simulink model "Boeing787_OldMission_ElectricalThermalHydraulicFuelECS"  (R2013a)
settings: Solver=ode23tb  SolverMode=SingleTasking  StartTime=0.0  StopTime=346  RelTol=1e-3
InitFcn:
  | load('SampleOutput.mat')
  | 
  | load('SampleFuelBurn.mat')
undefined symbols (not defined in the file or in its folder): ailerons, AirProp, B_737, elevator, FuelBurn, HydProp, landing_gear, rudder, thrust_rev
libraries: PowerFlowLib x118, simulink x20
(part 17 of 26)

== system Boeing787_OldMission_ElectricalThermalHydraulicFuelECS/Fuel ==
  note: Fuel & Oil System
  ECS : Inport
  Eng1 : Inport  Port=2
  Eng2 : Inport  Port=3  PortDimensions=11
  Bus Creator : BusCreator  Inputs=3
  Constant : Constant  Value=50
  Constant1 : Constant  Value=1700
  Constant2 : Constant  Value=1700
  Constant{3..6} (4 alike) : Constant  Value=0
  ElectricalSink : PowerFlowLib/Support Functions//Tools/ElectricalSink  Tag=Flow  Description=TwoPhase  load_loc=Empennage  ACDC_load=AC  units=Kilowatts  unq_id=2143
  ElectricalSink1 : PowerFlowLib/Support Functions//Tools/ElectricalSink  Tag=Flow  Description=TwoPhase  load_loc=Cagobay  ACDC_load=AC  units=Kilowatts  unq_id=9219
  ElectricalSink2 : PowerFlowLib/Support Functions//Tools/ElectricalSink  Tag=Flow  Description=TwoPhase  load_loc=Cabin  ACDC_load=AC  units=Kilowatts  unq_id=6691
  Fuel Tanks/Pumps : Subsystem
  Heat Exchanger : PowerFlowLib/Energy & Power Systems/Thermal/Fuel & Oil/Heat Exchanger  fld1=Oil  fld2=Air  Tw_init=90  C_wall=60000  Tw0=90  Q0=20000  H1_0=10000  A1=0.18984  mdot1_0=1.2  Tin1_0=105  Pin1_0=101  H2_0=10000  A2=0.045127  mdot2_0=1  Tin2_0=35  Pin2_0=50
  Heat Exchanger1 : PowerFlowLib/Energy & Power Systems/Thermal/Fuel & Oil/Heat Exchanger  fld1=Oil  fld2=Air  Tw_init=90  C_wall=60000  Tw0=90  Q0=20000  H1_0=10000  A1=0.18984  mdot1_0=1.2  Tin1_0=105  Pin1_0=101  H2_0=10000  A2=0.045127  mdot2_0=1  Tin2_0=35  Pin2_0=50
  Heat Exchanger2 : PowerFlowLib/Energy & Power Systems/Thermal/Fuel & Oil/Heat Exchanger  fld1=Oil  fld2=Fuel  Tw_init=80  C_wall=60000  Tw0=80  Q0=40000  H1_0=20000  A1=0.17164  mdot1_0=1  Tin1_0=55  Pin1_0=100  H2_0=20000  A2=0.53191  mdot2_0=1.2  Tin2_0=95  Pin2_0=101
  Heat Exchanger3 : PowerFlowLib/Energy & Power Systems/Thermal/Fuel & Oil/Heat Exchanger  fld1=Oil  fld2=Fuel  Tw_init=80  C_wall=60000  Tw0=80  Q0=40000  H1_0=20000  A1=0.17164  mdot1_0=1  Tin1_0=55  Pin1_0=100  H2_0=20000  A2=0.53191  mdot2_0=1.2  Tin2_0=95  Pin2_0=101
  Oil Tanks/Pumps Left Wing : Subsystem
  Oil Tanks/Pumps Right Wing : Subsystem
  Oil Left : Outport
  Fuel Left : Outport  Port=2
  Fuel Right : Outport  Port=3
  Oil Right : Outport  Port=4
  wires:
  Constant/1 -> Fuel Tanks/Pumps/1(Pamb)
  Heat Exchanger1/1 -> Heat Exchanger3/1
  Fuel Tanks/Pumps/2(Fuel Right Wing) -> Heat Exchanger3/2
  Oil Tanks/Pumps Right Wing/1(Oil To HX) -> Heat Exchanger1/1
  Constant1/1 -> Oil Tanks/Pumps Right Wing/1(Oil Sys Pres)
  Heat Exchanger3/2 -> Fuel Right/1  "Fuel_Right_Engine"
  Heat Exchanger/1 -> Heat Exchanger2/1
  Oil Tanks/Pumps Left Wing/1(Oil To HX) -> Heat Exchanger/1
  Constant2/1 -> Oil Tanks/Pumps Left Wing/1(Oil Sys Pres)
  Fuel Tanks/Pumps/1(Fuel Left Wing) -> Heat Exchanger2/2
  Heat Exchanger2/2 -> Fuel Left/1  "Fuel_Left_Engine"
  Heat Exchanger3/1 -> Oil Right/1  "Oil_Right_Engine"
  Constant3/1 -> ElectricalSink1/1, ElectricalSink2/1, ElectricalSink2/2, ElectricalSink1/2, ElectricalSink/1, ElectricalSink/2
  [Eng1] -> Oil Tanks/Pumps Left Wing/2(Flow In)
  [Eng1] -> Fuel Tanks/Pumps/3(Fuel Demand Left Wing)
  Heat Exchanger2/1 -> Oil Left/1  "Oil_Left_Engine"
  Bus Creator/1 -> Heat Exchanger1/2, Heat Exchanger/2
  Constant4/1 -> Bus Creator/1  "pres_kPa"
  Constant5/1 -> Bus Creator/2  "temp_K"
  Constant6/1 -> Bus Creator/3  "mdot_kgps"
  ECS/1 -> [ECS]
  Eng1/1 -> [Eng1]
  Eng2/1 -> [Eng2]
  [Eng2] -> Fuel Tanks/Pumps/2(Fuel Demand Right Wing)
  [Eng2] -> Oil Tanks/Pumps Right Wing/2(Flow In)

== system Boeing787_OldMission_ElectricalThermalHydraulicFuelECS/Hydraulic ==
  note: Left Engine Hydraulic System
  note: Right Engine Hydraulic System
  note: Center Electrical Hydraulic System
  ELEC : Inport
  Eng1 : Inport  Port=2
  Eng2 : Inport  Port=3
  Bus Creator : BusCreator  Inputs=1
  Bus Creator1 : BusCreator  Inputs=2
  Center Hydraulic System : Subsystem  mask{Hyd_Pump_Pres=34473.79, DC_Motor_RPM1=0, DC_Motor_RPM2=0}
      mask prompts: Hyd_Pump_Pres "Hyrdaulic Pump Pressure (kpa)"; DC_Motor_RPM1 "DC Motor RPM 1"; DC_Motor_RPM2 "DC Motor RPM 2"
  Constant : Constant  Value=1000
  Left Hydraulic System : Subsystem  mask{Hyd_Pump_Pres=34473.79, DC_Motor_RPM=30000}
      mask prompts: Hyd_Pump_Pres "Hyrdaulic Pump Pressure (kpa)"; DC_Motor_RPM "DC Motor RPM"
  Mission Profile : PowerFlowLib/Mission Profile/Mission Profile  mssn_check=off  mssn_prof=MSSN  del_P=0  del_T=0  del_rho=0  pres_msl=101.3  temp_msl=15  dens_msl=1.229
  Right Hydraulic System : Subsystem  mask{Hyd_Pump_Pres=34473.79, DC_Motor_RPM=30000}
      mask prompts: Hyd_Pump_Pres "Hyrdaulic Pump Pressure (kpa)"; DC_Motor_RPM "DC Motor RPM"
  Scope : Scope
      settings: YMin=-0.065338  YMax=-0.065338  SaveName=ScopeData39
  "Hydr " : Outport
  wires:
  Mission Profile/1 -> [Mission]
  [Mission] -> Right Hydraulic System/1(Mission)
  [Mission] -> Center Hydraulic System/1(Mission)
  [Mission] -> Left Hydraulic System/1(Mission)
  Eng2/1 -> Right Hydraulic System/3(Eng2)
  Left Hydraulic System/1(Shaft Torque Eng1) -> [Shaft_Torque_1]
  Right Hydraulic System/1(Shaft Torque Eng2) -> [Shaft_Torque_2]
  [Elec] -> Center Hydraulic System/2(Elec)
  [Elec] -> Left Hydraulic System/2(Elec)
  [Elec] -> Right Hydraulic System/2(Elec)
  Bus Creator/1 -> [Elec]
  ELEC/1 -> Bus Creator/1
  Eng1/1 -> Left Hydraulic System/3(Eng1)
  [Shaft_Torque_1] -> Bus Creator1/1  "Torque1_Nm"
  [Shaft_Torque_2] -> Bus Creator1/2  "Torque2_Nm"
  Bus Creator1/1 -> Scope/1, "Hydr "/1

== system Boeing787_OldMission_ElectricalThermalHydraulicFuelECS/ECS/Electrical Sink Cabin ==
  In1 : Inport

== system Boeing787_OldMission_ElectricalThermalHydraulicFuelECS/ECS/Left Pack ==
  note: Packs have 2 motors each
  Voltage : Inport
  Ambient : Inport  Port=2
  "Area " : Constant  Value=.03
  Bus Creator : BusCreator  Inputs=3
  Bus Selector : BusSelector  OutputSignals=temp_K,pres_kPa,rho_kgpm3,Mach
  Compressor : Subsystem  AncestorBlock=PowerFlowLib/Energy & Power Systems/Thermal/ECS/Compressor
      mask help: COMPRESSOR (ECS)
      mask init:
      | load AirProp
      | load CompProp
      mask Help:
      | Main Assumptions
      | 1. The Turbine and the compressor are coupled to each other (turbocharger).
      | 2. Maps are provided to compute the efficiency of the compressor.
      | 3. There is no heat transfer from the compressor to the surrounding.
      mask Display:
      | image(imread('compressor.png'))
      | port_label('input',1,'{ \bfFlow In}','texmode','on')
      | port_label('input',2,'{ \bfShaft Speed}','texmode','on');
      | 
      | 
      | port_label('output',1,'{\bfFlow Out}','texmode','on')
      | port_label('output',2,'{\bfComp. Work}','texmode','on')
  Compressor1 : PowerFlowLib/Energy & Power Systems/Thermal/ECS/Compressor
      link override "m and P ": Gain=1
  Constant1 : Constant  Value=44000
  Constant5 : Constant  Value=35000
  DC Speed Servo1 : Subsystem  AncestorBlock=PowerFlowLib/Energy & Power Systems/Electrical/Machines/DC Speed Servo  mask{Vf=280, Ra=0.05, La=0.9e-3, Rfsh=400, Lfsh=320, Lmsh=1.9, J=1.5}
      mask prompts: Vf "Field voltage (V)"; Ra "Armature resistance (Ohms)"; La "Armature inductance (H)"; Rfsh "Shunt field resistance (Ohms)"; Lfsh "Shunt field inductance (H)"; Lmsh "Mutual inductance (H)"; J "Rotor moment of inertia (Kgm^2)"
  DC Speed Servo2 : Subsystem  AncestorBlock=PowerFlowLib/Energy & Power Systems/Electrical/Machines/DC Speed Servo  mask{Vf=280, Ra=0.05, La=0.9e-3, Rfsh=400, Lfsh=320, Lmsh=1.9, J=1.5}
      mask prompts: Vf "Field voltage (V)"; Ra "Armature resistance (Ohms)"; La "Armature inductance (H)"; Rfsh "Shunt field resistance (Ohms)"; Lfsh "Shunt field inductance (H)"; Lmsh "Mutual inductance (H)"; J "Rotor moment of inertia (Kgm^2)"
  Primary HX (air-air) : Subsystem  AncestorBlock=PowerFlowLib/Energy & Power Systems/Thermal/ECS/Air-Air HX  mask(Air-Air Heat Exchanger){L_hx=0.2, W_hx=0.2, H_hx=0.2, t_p=0.0008, K_p=167, cp_hx=883, m_cm=16, l_fin=.005, t_fin=0.0002, s_fin=0.0015, h_fin=0.0095, K_n=167, eta_f=0.8, T_cm_0=50}
      mask prompts: L_hx "Length of HX in the flow direction [m]"; W_hx "Width of HX [m]"; H_hx "Height of HX [m]"; t_p "HX plate thickness [m]"; K_p "Thermal conductivity of the plates [W/m.K]"; cp_hx "Specific heat of the HX material [J/kg.K]"; m_cm "Mass of HX [kg]"; l_fin "Fin length [m]"; t_fin "Fin thickness [m]"; s_fin "Fin free flow width [m]"; h_fin "Fin free flow height [m]"; K_n "Thermal conductivity of the fin material [W/m.K]"; eta_f "Fin efficiency"; T_cm_0 "Initial_HX_core_temp_[C]"
      mask init:
      | load AirProp
      mask Help:
      | Main Assumptions:
      | 
      | 1. Rectangular offset-strip fin heat exchanger.
      | 2. Lumped parameter model.
      | 3. Constant user-defined efficiency.
      | 4. Number of passages is the same for both the cold and hot fluid passages (usually
      | one of the flows has 1 more passage to reduce ambient losses).
      | 5. Similar plate and fin geometries for both the hot and cold fluid sides (the
      | objective is to simplify modeling and reduce the number of input parameters needed).
      | 6. Neglect heat transfer from fin face
      | 7. Neglect conduction heat transfer in the fin and plate bases
      mask Display:
      | port_label('input',1,'{ \bfFlow In (Hot)}','texmode','on')
      | port_label('input',2,'{ \bfFlow In (Cold)}','texmode','on');
      | 
      | port_label('output',1,'{\bfFlow Out (Hot)}','texmode','on')
      | port_label('output',2,'{\bfFlow Out (Cold)}','texmode','on')
      | port_label('output',3,'{\bfMisc. Data}','texmode','on')
  Product : Product
  Product1 : Product  Inputs=3
  Rate Limiter : RateLimiter  RisingSlewLimit=.02  FallingSlewLimit=-.02  SampleTimeMode=inherited
  Rate Limiter1 : RateLimiter  RisingSlewLimit=.02  FallingSlewLimit=-.02  SampleTimeMode=inherited
  Saturation : Saturate  UpperLimit=40000  LowerLimit=10000
  Saturation1 : Saturate  UpperLimit=60000  LowerLimit=30000
  Saturation2 : Saturate  UpperLimit=.5  LowerLimit=.01
  Scope{1..15} (15 alike) : Scope
      Scope1 settings: YMin=469600  YMax=470800  SaveName=ScopeData6
      Scope10 settings: YMin=0  YMax=0.25  SaveName=ScopeData17
      Scope11 settings: YMin=-1750  YMax=500
      Scope12 settings: SaveName=ScopeData19
      Scope13 settings: YMin=0  YMax=750  SaveName=ScopeData2
      Scope14 settings: YMin=0  YMax=375  SaveName=ScopeData4
      Scope15 settings: YMin=0  YMax=300  SaveName=ScopeData5
      Scope2 settings: YMin=-2.5e+06  YMax=4e+06  SaveName=ScopeData7
      Scope3 settings: YMin=4.29e+06  YMax=4.3e+06  SaveName=ScopeData8
      Scope4 settings: SaveName=ScopeData9
      Scope5 settings: YMin=0  YMax=11000  SaveName=ScopeData10
      Scope6 settings: SaveName=ScopeData11
      Scope7 settings: TimeRange=10000  YMin=0  YMax=350  SaveName=ScopeData12
      Scope8 settings: YMin=0  YMax=850  SaveName=ScopeData13
      Scope9 settings: YMin=0  YMax=350  SaveName=ScopeData14
  Secondary HX (air-air)1 : Subsystem  AncestorBlock=PowerFlowLib/Energy & Power Systems/Thermal/ECS/Air-Air HX  mask(Air-Air Heat Exchanger){L_hx=0.2, W_hx=0.2, H_hx=0.2, t_p=0.0008, K_p=167, cp_hx=883, m_cm=16, l_fin=.005, t_fin=0.0002, s_fin=0.0015, h_fin=0.0095, K_n=167, eta_f=0.8, T_cm_0=50}
      mask prompts: L_hx "Length of HX in the flow direction [m]"; W_hx "Width of HX [m]"; H_hx "Height of HX [m]"; t_p "HX plate thickness [m]"; K_p "Thermal conductivity of the plates [W/m.K]"; cp_hx "Specific heat of the HX material [J/kg.K]"; m_cm "Mass of HX [kg]"; l_fin "Fin length [m]"; t_fin "Fin thickness [m]"; s_fin "Fin free flow width [m]"; h_fin "Fin free flow height [m]"; K_n "Thermal conductivity of the fin material [W/m.K]"; eta_f "Fin efficiency"; T_cm_0 "Initial_HX_core_temp_[C]"
      mask init:
      | load AirProp
      mask Help:
      | Main Assumptions:
      | 
      | 1. Rectangular offset-strip fin heat exchanger.
      | 2. Lumped parameter model.
      | 3. Constant user-defined efficiency.
      | 4. Number of passages is the same for both the cold and hot fluid passages (usually
      | one of the flows has 1 more passage to reduce ambient losses).
      | 5. Similar plate and fin geometries for both the hot and cold fluid sides (the
      | objective is to simplify modeling and reduce the number of input parameters needed).
      | 6. Neglect heat transfer from fin face
      | 7. Neglect conduction heat transfer in the fin and plate bases
      mask Display:
      | port_label('input',1,'{ \bfFlow In (Hot)}','texmode','on')
      | port_label('input',2,'{ \bfFlow In (Cold)}','texmode','on');
      | 
      | port_label('output',1,'{\bfFlow Out (Hot)}','texmode','on')
      | port_label('output',2,'{\bfFlow Out (Cold)}','texmode','on')
      | port_label('output',3,'{\bfMisc. Data}','texmode','on')
  Speed of Sound : Constant  Value=340
  Sum : Sum  Inputs=|++
  Terminator{,1..3,5} (5 alike) : Terminator
  Turbine : PowerFlowLib/Energy & Power Systems/Thermal/ECS/Turbine  press_Turbine_exit=80  inertia=5e-5  n_t=0.7
  Flow Out : Outport
  wires:
  [Voltage] -> DC Speed Servo1/3(Voltage)
  Constant5/1 -> Saturation/1
  DC Speed Servo1/1(w_m) -> Scope5/1, Compressor/2(In4)
  Compressor/1(Out1) -> Scope7/1, [Flow1]
  [RamAir_Left1] -> Scope6/1, Compressor/1(In2)
  Voltage/1 -> [Voltage]
  [Voltage] -> DC Speed Servo2/3(Voltage)
  Constant1/1 -> Saturation1/1
  DC Speed Servo2/1(w_m) -> Compressor1/2
  [Flow1] -> Scope9/1, Compressor1/1
  [RamAir_Left1] -> Primary HX (air-air)/2(In_flow_bus_cold)
  Compressor1/1 -> Scope8/1, Primary HX (air-air)/1(In_flow_bus_hot)
  ? -> [pHX_out2], Scope11/1
  Primary HX (air-air)/2(Out_flow_bus_cold) -> Terminator5/1
  Primary HX (air-air)/3(Other_outputs) -> Terminator1/1
  Primary HX (air-air)/1(Out_flow_bus_hot) -> Scope14/1, Secondary HX (air-air)1/1(In_flow_bus_hot), [pHX_out1]
  Turbine/2 -> [Shaft_speed]
  Turbine/1 -> Scope13/1, Flow Out/1, [turb_out]
  Ambient/1 -> Bus Selector/1
  [pHX_out1] -> Terminator/1
  Bus Creator/1 -> Scope15/1, [RamAir_Left1]
  Bus Selector/1 -> [Ambient_Temp_Left]  "<temp_K>"
  Saturation/1 -> DC Speed Servo1/2(Speed_ref (RPM))
  Saturation1/1 -> DC Speed Servo2/2(Speed_ref (RPM))
  Compressor/2(Power_out) -> [Torque1], Scope4/1
  [Torque1] -> DC Speed Servo1/1(T_load (Nm))
  Compressor1/2 -> Turbine/2, Scope1/1, Sum/1
  Sum/1 -> Scope3/1, [Torque2]
  [Torque2] -> DC Speed Servo2/1(T_load (Nm))
  Turbine/3 -> Sum/2, Scope2/1
  [Ambient_Temp_Left] -> Bus Creator/1  "temp_K"
  [Ambient_Pres_Left] -> Bus Creator/2  "pres_kPa"
  Product1/1 -> Rate Limiter1/1, Scope10/1  "mdot_kgps"
  Bus Selector/2 -> [Ambient_Pres_Left]  "<pres_kPa>"
  Bus Selector/3 -> [Ambient_Rho_Left]  "<rho_kgpm3>"
  Bus Selector/4 -> [Ambient_Mach_Left]  "<Mach>"
  Speed of Sound/1 -> Product/2
  [Ambient_Rho_Left] -> Product1/3
  Product/1 -> Product1/1, Scope12/1
  [Ambient_Mach_Left] -> Rate Limiter/1
  "Area "/1 -> Product1/2  "mdot_kgps"
  Saturation2/1 -> Bus Creator/3  "mdot_kgps"
  [turb_out] -> Secondary HX (air-air)1/2(In_flow_bus_cold)
  Secondary HX (air-air)1/1(Out_flow_bus_hot) -> Turbine/1
  Secondary HX (air-air)1/2(Out_flow_bus_cold) -> Terminator3/1
  Secondary HX (air-air)1/3(Other_outputs) -> Terminator2/1
  Rate Limiter/1 -> Product/1
  Rate Limiter1/1 -> Saturation2/1

== system Boeing787_OldMission_ElectricalThermalHydraulicFuelECS/ECS/Right Pack1 ==
  note: Packs have 2 motors each
  Voltage : Inport
  Ambient : Inport  Port=2
  "Area " : Constant  Value=.03
  Bus Creator : BusCreator  Inputs=3
  Bus Selector : BusSelector  OutputSignals=temp_K,pres_kPa,rho_kgpm3,Mach
  Compressor : Subsystem  AncestorBlock=PowerFlowLib/Energy & Power Systems/Thermal/ECS/Compressor
      mask help: COMPRESSOR (ECS)
      mask init:
      | load AirProp
      | load CompProp
      mask Help:
      | Main Assumptions
      | 1. The Turbine and the compressor are coupled to each other (turbocharger).
      | 2. Maps are provided to compute the efficiency of the compressor.
      | 3. There is no heat transfer from the compressor to the surrounding.
      mask Display:
      | image(imread('compressor.png'))
      | port_label('input',1,'{ \bfFlow In}','texmode','on')
      | port_label('input',2,'{ \bfShaft Speed}','texmode','on');
      | 
      | 
      | port_label('output',1,'{\bfFlow Out}','texmode','on')
      | port_label('output',2,'{\bfComp. Work}','texmode','on')
  Compressor1 : PowerFlowLib/Energy & Power Systems/Thermal/ECS/Compressor
      link override "m and P ": Gain=1
  Constant1 : Constant  Value=44000
  Constant5 : Constant  Value=35000
  DC Speed Servo1 : Subsystem  AncestorBlock=PowerFlowLib/Energy & Power Systems/Electrical/Machines/DC Speed Servo  mask{Vf=280, Ra=0.05, La=0.9e-3, Rfsh=400, Lfsh=320, Lmsh=1.9, J=1.5}
      mask prompts: Vf "Field voltage (V)"; Ra "Armature resistance (Ohms)"; La "Armature inductance (H)"; Rfsh "Shunt field resistance (Ohms)"; Lfsh "Shunt field inductance (H)"; Lmsh "Mutual inductance (H)"; J "Rotor moment of inertia (Kgm^2)"
  DC Speed Servo2 : Subsystem  AncestorBlock=PowerFlowLib/Energy & Power Systems/Electrical/Machines/DC Speed Servo  mask{Vf=280, Ra=0.05, La=0.9e-3, Rfsh=400, Lfsh=320, Lmsh=1.9, J=1.5}
      mask prompts: Vf "Field voltage (V)"; Ra "Armature resistance (Ohms)"; La "Armature inductance (H)"; Rfsh "Shunt field resistance (Ohms)"; Lfsh "Shunt field inductance (H)"; Lmsh "Mutual inductance (H)"; J "Rotor moment of inertia (Kgm^2)"
  Primary HX (air-air) : Subsystem  AncestorBlock=PowerFlowLib/Energy & Power Systems/Thermal/ECS/Air-Air HX  mask(Air-Air Heat Exchanger){L_hx=0.2, W_hx=0.2, H_hx=0.2, t_p=0.0008, K_p=167, cp_hx=883, m_cm=16, l_fin=.005, t_fin=0.0002, s_fin=0.0015, h_fin=0.0095, K_n=167, eta_f=0.8, T_cm_0=50}
      mask prompts: L_hx "Length of HX in the flow direction [m]"; W_hx "Width of HX [m]"; H_hx "Height of HX [m]"; t_p "HX plate thickness [m]"; K_p "Thermal conductivity of the plates [W/m.K]"; cp_hx "Specific heat of the HX material [J/kg.K]"; m_cm "Mass of HX [kg]"; l_fin "Fin length [m]"; t_fin "Fin thickness [m]"; s_fin "Fin free flow width [m]"; h_fin "Fin free flow height [m]"; K_n "Thermal conductivity of the fin material [W/m.K]"; eta_f "Fin efficiency"; T_cm_0 "Initial_HX_core_temp_[C]"
      mask init:
      | load AirProp
      mask Help:
      | Main Assumptions:
      | 
      | 1. Rectangular offset-strip fin heat exchanger.
      | 2. Lumped parameter model.
      | 3. Constant user-defined efficiency.
      | 4. Number of passages is the same for both the cold and hot fluid passages (usually
      | one of the flows has 1 more passage to reduce ambient losses).
      | 5. Similar plate and fin geometries for both the hot and cold fluid sides (the
      | objective is to simplify modeling and reduce the number of input parameters needed).
      | 6. Neglect heat transfer from fin face
      | 7. Neglect conduction heat transfer in the fin and plate bases
      mask Display:
      | port_label('input',1,'{ \bfFlow In (Hot)}','texmode','on')
      | port_label('input',2,'{ \bfFlow In (Cold)}','texmode','on');
      | 
      | port_label('output',1,'{\bfFlow Out (Hot)}','texmode','on')
      | port_label('output',2,'{\bfFlow Out (Cold)}','texmode','on')
      | port_label('output',3,'{\bfMisc. Data}','texmode','on')
  Product : Product
  Product1 : Product  Inputs=3
  Rate Limiter : RateLimiter  RisingSlewLimit=.02  FallingSlewLimit=-.02  SampleTimeMode=inherited
  Rate Limiter1 : RateLimiter  RisingSlewLimit=.02  FallingSlewLimit=-.02  SampleTimeMode=inherited
  Saturation : Saturate  UpperLimit=40000  LowerLimit=10000
  Saturation1 : Saturate  UpperLimit=60000  LowerLimit=30000
  Saturation2 : Saturate  UpperLimit=.5  LowerLimit=.01
  Scope{1..15} (15 alike) : Scope
      Scope1 settings: YMin=469600  YMax=470800  SaveName=ScopeData6
      Scope10 settings: YMin=0  YMax=0.25  SaveName=ScopeData17
      Scope11 settings: YMin=-1750  YMax=500
      Scope12 settings: SaveName=ScopeData19
      Scope13 settings: YMin=0  YMax=750  SaveName=ScopeData2
      Scope14 settings: YMin=0  YMax=375  SaveName=ScopeData4
      Scope15 settings: YMin=0  YMax=300  SaveName=ScopeData5
      Scope2 settings: YMin=-2.5e+06  YMax=4e+06  SaveName=ScopeData7
      Scope3 settings: YMin=4.29e+06  YMax=4.3e+06  SaveName=ScopeData8
      Scope4 settings: SaveName=ScopeData9
      Scope5 settings: YMin=0  YMax=11000  SaveName=ScopeData10
      Scope6 settings: SaveName=ScopeData11
      Scope7 settings: TimeRange=10000  YMin=0  YMax=350  SaveName=ScopeData12
      Scope8 settings: YMin=0  YMax=850  SaveName=ScopeData13
      Scope9 settings: YMin=0  YMax=350  SaveName=ScopeData14
  Secondary HX (air-air)1 : Subsystem  AncestorBlock=PowerFlowLib/Energy & Power Systems/Thermal/ECS/Air-Air HX  mask(Air-Air Heat Exchanger){L_hx=0.2, W_hx=0.2, H_hx=0.2, t_p=0.0008, K_p=167, cp_hx=883, m_cm=16, l_fin=.005, t_fin=0.0002, s_fin=0.0015, h_fin=0.0095, K_n=167, eta_f=0.8, T_cm_0=50}
      mask prompts: L_hx "Length of HX in the flow direction [m]"; W_hx "Width of HX [m]"; H_hx "Height of HX [m]"; t_p "HX plate thickness [m]"; K_p "Thermal conductivity of the plates [W/m.K]"; cp_hx "Specific heat of the HX material [J/kg.K]"; m_cm "Mass of HX [kg]"; l_fin "Fin length [m]"; t_fin "Fin thickness [m]"; s_fin "Fin free flow width [m]"; h_fin "Fin free flow height [m]"; K_n "Thermal conductivity of the fin material [W/m.K]"; eta_f "Fin efficiency"; T_cm_0 "Initial_HX_core_temp_[C]"
      mask init:
      | load AirProp
      mask Help:
      | Main Assumptions:
      | 
      | 1. Rectangular offset-strip fin heat exchanger.
      | 2. Lumped parameter model.
      | 3. Constant user-defined efficiency.
      | 4. Number of passages is the same for both the cold and hot fluid passages (usually
      | one of the flows has 1 more passage to reduce ambient losses).
      | 5. Similar plate and fin geometries for both the hot and cold fluid sides (the
      | objective is to simplify modeling and reduce the number of input parameters needed).
      | 6. Neglect heat transfer from fin face
      | 7. Neglect conduction heat transfer in the fin and plate bases
      mask Display:
      | port_label('input',1,'{ \bfFlow In (Hot)}','texmode','on')
      | port_label('input',2,'{ \bfFlow In (Cold)}','texmode','on');
      | 
      | port_label('output',1,'{\bfFlow Out (Hot)}','texmode','on')
      | port_label('output',2,'{\bfFlow Out (Cold)}','texmode','on')
      | port_label('output',3,'{\bfMisc. Data}','texmode','on')
  Speed of Sound : Constant  Value=340
  Sum : Sum  Inputs=|++
  Terminator{,1..3,5} (5 alike) : Terminator
  Turbine : PowerFlowLib/Energy & Power Systems/Thermal/ECS/Turbine  press_Turbine_exit=80  inertia=5e-5  n_t=0.7
  Flow Out : Outport
  wires:
  [Voltage] -> DC Speed Servo1/3(Voltage)
  Constant5/1 -> Saturation/1
  DC Speed Servo1/1(w_m) -> Scope5/1, Compressor/2(In4)
  Compressor/1(Out1) -> Scope7/1, [Flow1]
  [RamAir_Left1] -> Scope6/1, Compressor/1(In2)
  Voltage/1 -> [Voltage]
  [Voltage] -> DC Speed Servo2/3(Voltage)
  Constant1/1 -> Saturation1/1
  DC Speed Servo2/1(w_m) -> Compressor1/2
  [Flow1] -> Scope9/1, Compressor1/1
  [RamAir_Left1] -> Primary HX (air-air)/2(In_flow_bus_cold)
  Compressor1/1 -> Scope8/1, Primary HX (air-air)/1(In_flow_bus_hot)
  ? -> [pHX_out2], Scope11/1
  Primary HX (air-air)/2(Out_flow_bus_cold) -> Terminator5/1
  Primary HX (air-air)/3(Other_outputs) -> Terminator1/1
  Primary HX (air-air)/1(Out_flow_bus_hot) -> Scope14/1, Secondary HX (air-air)1/1(In_flow_bus_hot), [pHX_out1]
  Turbine/2 -> [Shaft_speed]
  Turbine/1 -> Scope13/1, Flow Out/1, [turb_out]
  Ambient/1 -> Bus Selector/1
  [pHX_out1] -> Terminator/1
  Bus Creator/1 -> Scope15/1, [RamAir_Left1]
  Bus Selector/1 -> [Ambient_Temp_Left]  "<temp_K>"
  Saturation/1 -> DC Speed Servo1/2(Speed_ref (RPM))
  Saturation1/1 -> DC Speed Servo2/2(Speed_ref (RPM))
  Compressor/2(Power_out) -> [Torque1], Scope4/1
  [Torque1] -> DC Speed Servo1/1(T_load (Nm))
  Compressor1/2 -> Turbine/2, Scope1/1, Sum/1
  Sum/1 -> Scope3/1, [Torque2]
  [Torque2] -> DC Speed Servo2/1(T_load (Nm))
  Turbine/3 -> Sum/2, Scope2/1
  [Ambient_Temp_Left] -> Bus Creator/1  "temp_K"
  [Ambient_Pres_Left] -> Bus Creator/2  "pres_kPa"
  Product1/1 -> Rate Limiter1/1, Scope10/1  "mdot_kgps"
  Bus Selector/2 -> [Ambient_Pres_Left]  "<pres_kPa>"
  Bus Selector/3 -> [Ambient_Rho_Left]  "<rho_kgpm3>"
  Bus Selector/4 -> [Ambient_Mach_Left]  "<Mach>"
  Speed of Sound/1 -> Product/2
  [Ambient_Rho_Left] -> Product1/3
  Product/1 -> Product1/1, Scope12/1
  [Ambient_Mach_Left] -> Rate Limiter/1
  "Area "/1 -> Product1/2  "mdot_kgps"
  Saturation2/1 -> Bus Creator/3  "mdot_kgps"
  [turb_out] -> Secondary HX (air-air)1/2(In_flow_bus_cold)
  Secondary HX (air-air)1/1(Out_flow_bus_hot) -> Turbine/1
  Secondary HX (air-air)1/2(Out_flow_bus_cold) -> Terminator3/1
  Secondary HX (air-air)1/3(Other_outputs) -> Terminator2/1
  Rate Limiter/1 -> Product/1
  Rate Limiter1/1 -> Saturation2/1

== system Boeing787_OldMission_ElectricalThermalHydraulicFuelECS/ECS/Thermal Loads ==
  "Thermal Loads " : Outport

== system Boeing787_OldMission_ElectricalThermalHydraulicFuelECS/Electrical/230 Vac Distr ==
  note: Generator Bus 1
  note: Generator Bus 2
  Gen 1 : Inport
  Gen 2 : Inport  Port=2
  Gen 3 : Inport  Port=3
  Gen 4 : Inport  Port=4
  Gen 5 : Inport  Port=5
  Gen 6 : Inport  Port=6
  I_Bus : Inport  Port=7
  Gain : Gain  Gain=1/2
  Gen Bus w/ APU switch : PowerFlowLib/Energy & Power Systems/Electrical/Systems/Gen Bus w// APU switch  LOWVLIMIT=90  UPVLIMIT=250  bus_st=2
  Gen Bus w/ APU switch1 : PowerFlowLib/Energy & Power Systems/Electrical/Systems/Gen Bus w// APU switch  LOWVLIMIT=90  UPVLIMIT=250  bus_st=2
  Terminator : Terminator
  Terminator1 : Terminator
  Vbus1 : Outport
  Vbus2 : Outport  Port=2
  tag scope: i_APU1=global, i_APU2=global, i_GND1=global, i_GND2=global, i_MAIN1=global, i_MAIN2=global
  wires:
  Gen Bus w/ APU switch/3 -> [i_APU1]
  Gen Bus w/ APU switch/4 -> [i_GND1]
  [Gen_Bus1] -> Gen Bus w/ APU switch/1
  Gen Bus w/ APU switch/2 -> [i_MAIN1]
  Gen Bus w/ APU switch1/3 -> [i_APU2]
  Gen Bus w/ APU switch1/4 -> [i_GND2]
  Gen Bus w/ APU switch1/2 -> [i_MAIN2]
  [Gen_Bus2] -> Gen Bus w/ APU switch1/1
  Gen 1/1 -> Gen Bus w/ APU switch/2
  Gen 3/1 -> Gen Bus w/ APU switch1/2
  Gen 5/1 -> Gen Bus w/ APU switch/3
  Gen 6/1 -> Gen Bus w/ APU switch1/3
  Gen Bus w/ APU switch/1 -> Vbus1/1
  Gen Bus w/ APU switch1/1 -> Vbus2/1
  I_Bus/1 -> Gain/1
  Gain/1 -> Gen Bus w/ APU switch1/6, Gen Bus w/ APU switch/6
  Gen 2/1 -> Terminator/1
  Gen 4/1 -> Terminator1/1

== system Boeing787_OldMission_ElectricalThermalHydraulicFuelECS/Electrical/Automatic Transformer Rectifier Unit ==
  Vin dqo : Inport
  Iout dqo : Inport  Port=2
  Constant : Constant  Value=[0.5 0.5 0.5]
  Demux : Demux  Outputs=3
  Demux1 : Demux  Outputs=3
  Gain : Gain  Gain=.5
  Mux1 : Mux  Inputs=3
  Mux2 : Mux  Inputs=3
  Three Phase Full Bridge Practical : PowerFlowLib/Energy & Power Systems/Electrical/Rectifiers/Three Phase Full Bridge Practical  C=100e-6  Rc=1
  abc to qd0 : PowerFlowLib/Energy & Power Systems/Electrical/Coordinate Transformation/abc to qd0
  qd0 to abc : PowerFlowLib/Energy & Power Systems/Electrical/Coordinate Transformation/qd0 to abc
  three-phase full-bridge inverter1 : PowerFlowLib/Energy & Power Systems/Electrical/Inverters/three-phase  full-bridge  inverter1
  Vout dqo : Outport
  Iin : Outport  Port=2
  wires:
  Three Phase Full Bridge Practical/1 -> three-phase full-bridge inverter1/2
  Constant/1 -> three-phase full-bridge inverter1/1
  three-phase full-bridge inverter1/1 -> Demux/1
  Demux/1 -> abc to qd0/1
  Demux/2 -> abc to qd0/2
  Demux/3 -> abc to qd0/3
  abc to qd0/1 -> Mux1/1
  abc to qd0/2 -> Mux1/2
  abc to qd0/3 -> Mux1/3
  three-phase full-bridge inverter1/2 -> Three Phase Full Bridge Practical/2
  Demux1/1 -> qd0 to abc/1
  Demux1/2 -> qd0 to abc/2
  Demux1/3 -> qd0 to abc/3
  qd0 to abc/1 -> Mux2/1
  qd0 to abc/2 -> Mux2/2
  qd0 to abc/3 -> Mux2/3
  Mux2/1 -> three-phase full-bridge inverter1/3
  Three Phase Full Bridge Practical/2 -> Iin/1
  Iout dqo/1 -> Demux1/1
  Vin dqo/1 -> Three Phase Full Bridge Practical/1
  Mux1/1 -> Gain/1
  Gain/1 -> Vout dqo/1

== system Boeing787_OldMission_ElectricalThermalHydraulicFuelECS/Electrical/Bus Controls ==
  Constant{1..5} (5 alike) : Constant
  Gen_Bus1 : Outport
  Gen_Bus2 : Outport  Port=2
  270V_DC_Bus : Outport  Port=3
  115V_AC_Bus : Outport  Port=4
  28V_DC_Bus : Outport  Port=5
  wires:
  Constant3/1 -> 28V_DC_Bus/1
  Constant5/1 -> 115V_AC_Bus/1
  Constant2/1 -> 270V_DC_Bus/1
  Constant4/1 -> Gen_Bus2/1
  Constant1/1 -> Gen_Bus1/1

== system Boeing787_OldMission_ElectricalThermalHydraulicFuelECS/Electrical/DC Bus 1 ==
  Select : Inport
  VDC_1 : Inport  Port=2
  VDC_2 : Inport  Port=3
  Load current : Inport  Port=4
  Compare To Constant : simulink/Logic and Bit Operations/Compare To Constant  relop=<=  const=3.0  OutDataTypeStr=boolean
  Compare To Constant1 : simulink/Logic and Bit Operations/Compare To Constant  relop=<=  const=3.0  OutDataTypeStr=boolean
  Constant : Constant  Value=[0]
  Multiport Switch : MultiPortSwitch  Inputs=2
  Switch : Switch  Criteria=u2 ~= 0
  Switch1 : Switch  Criteria=u2 ~= 0
  Vbus : Outport
  IDC_1 : Outport  Port=2
  IDC_2 : Outport  Port=3
  wires:
  Load current/1 -> Switch1/1, Switch/1
  Multiport Switch/1 -> Vbus/1
  VDC_1/1 -> Multiport Switch/2
  VDC_2/1 -> Multiport Switch/3
  Select/1 -> Multiport Switch/1, Compare To Constant/1, Compare To Constant1/1
  Compare To Constant/1 -> Switch/2
  Compare To Constant1/1 -> Switch1/2
  Constant/1 -> Switch/3, Switch1/3
  Switch/1 -> IDC_1/1
  Switch1/1 -> IDC_2/1

== system Boeing787_OldMission_ElectricalThermalHydraulicFuelECS/Electrical/DC Bus 3 ==
  Select : Inport
  VDC_1 : Inport  Port=2
  VDC_2 : Inport  Port=3
  Load current : Inport  Port=4
  Compare To Constant : simulink/Logic and Bit Operations/Compare To Constant  relop=<=  const=3.0  OutDataTypeStr=boolean
  Compare To Constant1 : simulink/Logic and Bit Operations/Compare To Constant  relop=<=  const=3.0  OutDataTypeStr=boolean
  Constant : Constant  Value=[0]
  Multiport Switch : MultiPortSwitch  Inputs=2
  Switch : Switch  Criteria=u2 ~= 0
  Switch1 : Switch  Criteria=u2 ~= 0
  Vbus : Outport
  IDC_1 : Outport  Port=2
  IDC_2 : Outport  Port=3
  wires:
  Load current/1 -> Switch1/1, Switch/1
  Multiport Switch/1 -> Vbus/1
  VDC_1/1 -> Multiport Switch/2
  VDC_2/1 -> Multiport Switch/3
  Select/1 -> Multiport Switch/1, Compare To Constant/1, Compare To Constant1/1
  Compare To Constant/1 -> Switch/2
  Compare To Constant1/1 -> Switch1/2
  Constant/1 -> Switch/3, Switch1/3
  Switch/1 -> IDC_1/1
  Switch1/1 -> IDC_2/1

== system Boeing787_OldMission_ElectricalThermalHydraulicFuelECS/Electrical/Enabled_AC_Loadloss ==
  Load Master Vector : Inport
  Vdq0 : Inport  Port=2
  Enable : EnablePort
  Enabled Subsystem : Subsystem  TreatAsAtomicUnit=on
  Enabled Subsystem1 : Subsystem  TreatAsAtomicUnit=on
  Sum1 : Sum  Inputs=|++
  Idq0 : Outport
  loss : Outport  Port=2
  wires:
  Enabled Subsystem/2(loss) -> loss/1
  Load Master Vector/1 -> Enabled Subsystem1/2(Ext vector)
  Sum1/1 -> Idq0/1
  Enabled Subsystem/1(Idq0) -> Sum1/2
  Enabled Subsystem1/1(Idq0) -> Sum1/1
  Vdq0/1 -> Enabled Subsystem1/1("Vdq0 "), Enabled Subsystem/1("Vdq0 ")

== system Boeing787_OldMission_ElectricalThermalHydraulicFuelECS/Electrical/Generation Unit Sync-Sync1 ==
  engine speed : Inport
  idq0 : Inport  Port=2
  Temperature : Inport  Port=3
  Bus Creator : BusCreator  Inputs=3
  Bus Creator1 : BusCreator  Inputs=3
  Coeff of Resistance : Gain  Gain=3.85e-3
  Demux : Demux  Outputs=3
  Gain : Gain  Gain=200*2/3
  Gain1 : Gain  Gain=200
  Generator : Subsystem
      mask Display:
      | p = 0:0.1:(2*pi+0.1);
      | plot(sin(p), cos(p));
      | p1 = (-pi/8-0.1-0.2):0.1:(pi/8+0.1-0.2);
      | plot(0.8*sin(p1), 0.8*cos(p1), 0.8*sin(p1+pi), 0.8*cos(p1+pi));
      | p2 = sin((-pi/8-0.1-0.2+pi/8+0.1-0.2)/2);
      | p3 = sin((-pi/8-0.1-0.2+pi/8+0.1-0.2)/2+pi);
      | p4 = cos((-pi/8-0.1-0.2+pi/8+0.1-0.2)/2);
      | p5 = cos((-pi/8-0.1-0.2+pi/8+0.1-0.2)/2+pi);
      | plot(0.8*[p2, p3], 0.8*[p4, p5]);
      | port_label('output', 1, 'Vdq0');
      | port_label('output', 2, 'Te');
      | port_label('output', 3, 'Vfd');
      | port_label('output', 4, 'Ploss');
      | port_label('input', 1, 'idq0');
      | port_label('input', 2, 'w');
      | port_label('input', 3, 'ifd');
  Initial Temperature : Constant  Value=25
  Memory : Memory
  Permanent Magnet Synchronous Generator1 : PowerFlowLib/Energy & Power Systems/Electrical/Machines/Permanent Magnet Synchronous Generator1
  RPM_to_radps : Gain  Gain=pi/30
  Scope2 : Scope
      settings: TimeRange=100  YMin=0  YMax=5500
  Sum : Sum  Inputs=++|
  Sum1 : Sum
  Sum5 : Sum  Inputs=|+-
  Sum6 : Sum  Inputs=|++
  control1 : Constant
  data_sink : PowerFlowLib/Support Functions//Tools/data_sink
  one : Constant
  three-phase active rectifier Voltage Mode : PowerFlowLib/Energy & Power Systems/Electrical/Rectifiers/three-phase  active rectifier Voltage Mode  L=1  C=1e-4
  vdq0 : Outport
  engine torque : Outport  Port=2
  Ploss : Outport  Port=3
  wires:
  Temperature/1 -> Sum5/1
  Initial Temperature/1 -> Sum5/2
  Sum5/1 -> Coeff of Resistance/1
  Coeff of Resistance/1 -> Sum6/1
  one/1 -> Sum6/2
  Sum6/1 -> [R_temp_delta]
  Memory/1 -> Permanent Magnet Synchronous Generator1/1
  Sum1/1 -> Ploss/1, Bus Creator/2  "Ploss (W)"
  Generator/4(Ploss) -> Sum1/2
  Permanent Magnet Synchronous Generator1/3 -> Sum1/1
  Generator/1(vdq0) -> vdq0/1, Demux/1  "Vdq0 (V)"
  idq0/1 -> Generator/1(idq0)
  Generator/2(Te) -> Sum/2
  Permanent Magnet Synchronous Generator1/2 -> Sum/1
  three-phase active rectifier Voltage Mode/2 -> Memory/1
  three-phase active rectifier Voltage Mode/1 -> Gain/1
  Gain/1 -> Bus Creator/3, Generator/3(ifd')  "Excit current (A)"
  Gain1/1 -> three-phase active rectifier Voltage Mode/3
  Generator/3(vfd') -> Gain1/1
  control1/1 -> three-phase active rectifier Voltage Mode/2
  Permanent Magnet Synchronous Generator1/1 -> three-phase active rectifier Voltage Mode/1
  RPM_to_radps/1 -> Permanent Magnet Synchronous Generator1/2, Generator/2(w), Scope2/1
  Sum/1 -> engine torque/1
  Bus Creator/1 -> data_sink/1
  Demux/1 -> Bus Creator1/1  "vd"
  Demux/2 -> Bus Creator1/2  "vq"
  Demux/3 -> Bus Creator1/3  "v0"
  Bus Creator1/1 -> Bus Creator/1  "vdq0 (V)"
  engine speed/1 -> RPM_to_radps/1
  [R_temp_delta] -> Generator/4(Temp)

== system Boeing787_OldMission_ElectricalThermalHydraulicFuelECS/Electrical/Generation Unit Sync-Sync2 ==
  engine speed : Inport
  idq0 : Inport  Port=2
  Temperature : Inport  Port=3
  Bus Creator : BusCreator  Inputs=3
  Bus Creator1 : BusCreator  Inputs=3
  Coeff of Resistance : Gain  Gain=3.85e-3
  Demux : Demux  Outputs=3
  Gain : Gain  Gain=200*2/3
  Gain1 : Gain  Gain=200
  Generator : Subsystem
      mask Display:
      | p = 0:0.1:(2*pi+0.1);
      | plot(sin(p), cos(p));
      | p1 = (-pi/8-0.1-0.2):0.1:(pi/8+0.1-0.2);
      | plot(0.8*sin(p1), 0.8*cos(p1), 0.8*sin(p1+pi), 0.8*cos(p1+pi));
      | p2 = sin((-pi/8-0.1-0.2+pi/8+0.1-0.2)/2);
      | p3 = sin((-pi/8-0.1-0.2+pi/8+0.1-0.2)/2+pi);
      | p4 = cos((-pi/8-0.1-0.2+pi/8+0.1-0.2)/2);
      | p5 = cos((-pi/8-0.1-0.2+pi/8+0.1-0.2)/2+pi);
      | plot(0.8*[p2, p3], 0.8*[p4, p5]);
      | port_label('output', 1, 'Vdq0');
      | port_label('output', 2, 'Te');
      | port_label('output', 3, 'Vfd');
      | port_label('output', 4, 'Ploss');
      | port_label('input', 1, 'idq0');
      | port_label('input', 2, 'w');
      | port_label('input', 3, 'ifd');
  Initial Temperature : Constant  Value=25
  Memory : Memory
  Permanent Magnet Synchronous Generator1 : PowerFlowLib/Energy & Power Systems/Electrical/Machines/Permanent Magnet Synchronous Generator1
  RPM_to_radps : Gain  Gain=pi/30
  Scope2 : Scope
      settings: TimeRange=100  YMin=0  YMax=5500
  Sum : Sum  Inputs=++|
  Sum1 : Sum
  Sum5 : Sum  Inputs=|+-
  Sum6 : Sum  Inputs=|++
  control1 : Constant
  data_sink : PowerFlowLib/Support Functions//Tools/data_sink
  one : Constant
  three-phase active rectifier Voltage Mode : PowerFlowLib/Energy & Power Systems/Electrical/Rectifiers/three-phase  active rectifier Voltage Mode  L=1  C=1e-4
  vdq0 : Outport
  engine torque : Outport  Port=2
  Ploss : Outport  Port=3
  wires:
  Temperature/1 -> Sum5/1
  Initial Temperature/1 -> Sum5/2
  Sum5/1 -> Coeff of Resistance/1
  Coeff of Resistance/1 -> Sum6/1
  one/1 -> Sum6/2
  Sum6/1 -> [R_temp_delta]
  Memory/1 -> Permanent Magnet Synchronous Generator1/1
  Sum1/1 -> Ploss/1, Bus Creator/2  "Ploss (W)"
  Generator/4(Ploss) -> Sum1/2
  Permanent Magnet Synchronous Generator1/3 -> Sum1/1
  Generator/1(vdq0) -> vdq0/1, Demux/1  "Vdq0 (V)"
  idq0/1 -> Generator/1(idq0)
  Generator/2(Te) -> Sum/2
  Permanent Magnet Synchronous Generator1/2 -> Sum/1
  three-phase active rectifier Voltage Mode/2 -> Memory/1
  three-phase active rectifier Voltage Mode/1 -> Gain/1
  Gain/1 -> Bus Creator/3, Generator/3(ifd')  "Excit current (A)"
  Gain1/1 -> three-phase active rectifier Voltage Mode/3
  Generator/3(vfd') -> Gain1/1
  control1/1 -> three-phase active rectifier Voltage Mode/2
  Permanent Magnet Synchronous Generator1/1 -> three-phase active rectifier Voltage Mode/1
  RPM_to_radps/1 -> Permanent Magnet Synchronous Generator1/2, Generator/2(w), Scope2/1
  Sum/1 -> engine torque/1
  Bus Creator/1 -> data_sink/1
  Demux/1 -> Bus Creator1/1  "vd"
  Demux/2 -> Bus Creator1/2  "vq"
  Demux/3 -> Bus Creator1/3  "v0"
  Bus Creator1/1 -> Bus Creator/1  "vdq0 (V)"
  engine speed/1 -> RPM_to_radps/1
  [R_temp_delta] -> Generator/4(Temp)

== system Boeing787_OldMission_ElectricalThermalHydraulicFuelECS/Electrical/Generation Unit Sync-Sync3 ==
  engine speed : Inport
  idq0 : Inport  Port=2
  Temperature : Inport  Port=3
  Bus Creator : BusCreator  Inputs=3
  Bus Creator1 : BusCreator  Inputs=3
  Coeff of Resistance : Gain  Gain=3.85e-3
  Demux : Demux  Outputs=3
  Gain : Gain  Gain=200*2/3
  Gain1 : Gain  Gain=200
  Generator : Subsystem
      mask Display:
      | p = 0:0.1:(2*pi+0.1);
      | plot(sin(p), cos(p));
      | p1 = (-pi/8-0.1-0.2):0.1:(pi/8+0.1-0.2);
      | plot(0.8*sin(p1), 0.8*cos(p1), 0.8*sin(p1+pi), 0.8*cos(p1+pi));
      | p2 = sin((-pi/8-0.1-0.2+pi/8+0.1-0.2)/2);
      | p3 = sin((-pi/8-0.1-0.2+pi/8+0.1-0.2)/2+pi);
      | p4 = cos((-pi/8-0.1-0.2+pi/8+0.1-0.2)/2);
      | p5 = cos((-pi/8-0.1-0.2+pi/8+0.1-0.2)/2+pi);
      | plot(0.8*[p2, p3], 0.8*[p4, p5]);
      | port_label('output', 1, 'Vdq0');
      | port_label('output', 2, 'Te');
      | port_label('output', 3, 'Vfd');
      | port_label('output', 4, 'Ploss');
      | port_label('input', 1, 'idq0');
      | port_label('input', 2, 'w');
      | port_label('input', 3, 'ifd');
  Initial Temperature : Constant  Value=25
  Memory : Memory
  Permanent Magnet Synchronous Generator1 : PowerFlowLib/Energy & Power Systems/Electrical/Machines/Permanent Magnet Synchronous Generator1
  RPM_to_radps : Gain  Gain=pi/30
  Scope2 : Scope
      settings: TimeRange=100  YMin=0  YMax=5500
  Sum : Sum  Inputs=++|
  Sum1 : Sum
  Sum5 : Sum  Inputs=|+-
  Sum6 : Sum  Inputs=|++
  control1 : Constant
  data_sink : PowerFlowLib/Support Functions//Tools/data_sink
  one : Constant
  three-phase active rectifier Voltage Mode : PowerFlowLib/Energy & Power Systems/Electrical/Rectifiers/three-phase  active rectifier Voltage Mode  L=1  C=1e-4
  vdq0 : Outport
  engine torque : Outport  Port=2
  Ploss : Outport  Port=3
  wires:
  Temperature/1 -> Sum5/1
  Initial Temperature/1 -> Sum5/2
  Sum5/1 -> Coeff of Resistance/1
  Coeff of Resistance/1 -> Sum6/1
  one/1 -> Sum6/2
  Sum6/1 -> [R_temp_delta]
  Memory/1 -> Permanent Magnet Synchronous Generator1/1
  Sum1/1 -> Ploss/1, Bus Creator/2  "Ploss (W)"
  Generator/4(Ploss) -> Sum1/2
  Permanent Magnet Synchronous Generator1/3 -> Sum1/1
  Generator/1(vdq0) -> vdq0/1, Demux/1  "Vdq0 (V)"
  idq0/1 -> Generator/1(idq0)
  Generator/2(Te) -> Sum/2
  Permanent Magnet Synchronous Generator1/2 -> Sum/1
  three-phase active rectifier Voltage Mode/2 -> Memory/1
  three-phase active rectifier Voltage Mode/1 -> Gain/1
  Gain/1 -> Bus Creator/3, Generator/3(ifd')  "Excit current (A)"
  Gain1/1 -> three-phase active rectifier Voltage Mode/3
  Generator/3(vfd') -> Gain1/1
  control1/1 -> three-phase active rectifier Voltage Mode/2
  Permanent Magnet Synchronous Generator1/1 -> three-phase active rectifier Voltage Mode/1
  RPM_to_radps/1 -> Permanent Magnet Synchronous Generator1/2, Generator/2(w), Scope2/1
  Sum/1 -> engine torque/1
  Bus Creator/1 -> data_sink/1
  Demux/1 -> Bus Creator1/1  "vd"
  Demux/2 -> Bus Creator1/2  "vq"
  Demux/3 -> Bus Creator1/3  "v0"
  Bus Creator1/1 -> Bus Creator/1  "vdq0 (V)"
  engine speed/1 -> RPM_to_radps/1
  [R_temp_delta] -> Generator/4(Temp)

== system Boeing787_OldMission_ElectricalThermalHydraulicFuelECS/Electrical/Generation Unit Sync-Sync4 ==
  engine speed : Inport
  idq0 : Inport  Port=2
  Temperature : Inport  Port=3
  Bus Creator : BusCreator  Inputs=3
  Bus Creator1 : BusCreator  Inputs=3
  Coeff of Resistance : Gain  Gain=3.85e-3
  Demux : Demux  Outputs=3
  Gain : Gain  Gain=200*2/3
  Gain1 : Gain  Gain=200
  Generator : Subsystem
      mask Display:
      | p = 0:0.1:(2*pi+0.1);
      | plot(sin(p), cos(p));
      | p1 = (-pi/8-0.1-0.2):0.1:(pi/8+0.1-0.2);
      | plot(0.8*sin(p1), 0.8*cos(p1), 0.8*sin(p1+pi), 0.8*cos(p1+pi));
      | p2 = sin((-pi/8-0.1-0.2+pi/8+0.1-0.2)/2);
      | p3 = sin((-pi/8-0.1-0.2+pi/8+0.1-0.2)/2+pi);
      | p4 = cos((-pi/8-0.1-0.2+pi/8+0.1-0.2)/2);
      | p5 = cos((-pi/8-0.1-0.2+pi/8+0.1-0.2)/2+pi);
      | plot(0.8*[p2, p3], 0.8*[p4, p5]);
      | port_label('output', 1, 'Vdq0');
      | port_label('output', 2, 'Te');
      | port_label('output', 3, 'Vfd');
      | port_label('output', 4, 'Ploss');
      | port_label('input', 1, 'idq0');
      | port_label('input', 2, 'w');
      | port_label('input', 3, 'ifd');
  Initial Temperature : Constant  Value=25
  Memory : Memory
  Permanent Magnet Synchronous Generator1 : PowerFlowLib/Energy & Power Systems/Electrical/Machines/Permanent Magnet Synchronous Generator1
  RPM_to_radps : Gain  Gain=pi/30
  Scope2 : Scope
      settings: TimeRange=100  YMin=0  YMax=5500
  Sum : Sum  Inputs=++|
  Sum1 : Sum
  Sum5 : Sum  Inputs=|+-
  Sum6 : Sum  Inputs=|++
  control1 : Constant
  data_sink : PowerFlowLib/Support Functions//Tools/data_sink
  one : Constant
  three-phase active rectifier Voltage Mode : PowerFlowLib/Energy & Power Systems/Electrical/Rectifiers/three-phase  active rectifier Voltage Mode  L=1  C=1e-4
  vdq0 : Outport
  engine torque : Outport  Port=2
  Ploss : Outport  Port=3
  wires:
  Temperature/1 -> Sum5/1
  Initial Temperature/1 -> Sum5/2
  Sum5/1 -> Coeff of Resistance/1
  Coeff of Resistance/1 -> Sum6/1
  one/1 -> Sum6/2
  Sum6/1 -> [R_temp_delta]
  Memory/1 -> Permanent Magnet Synchronous Generator1/1
  Sum1/1 -> Ploss/1, Bus Creator/2  "Ploss (W)"
  Generator/4(Ploss) -> Sum1/2
  Permanent Magnet Synchronous Generator1/3 -> Sum1/1
  Generator/1(vdq0) -> vdq0/1, Demux/1  "Vdq0 (V)"
  idq0/1 -> Generator/1(idq0)
  Generator/2(Te) -> Sum/2
  Permanent Magnet Synchronous Generator1/2 -> Sum/1
  three-phase active rectifier Voltage Mode/2 -> Memory/1
  three-phase active rectifier Voltage Mode/1 -> Gain/1
  Gain/1 -> Bus Creator/3, Generator/3(ifd')  "Excit current (A)"
  Gain1/1 -> three-phase active rectifier Voltage Mode/3
  Generator/3(vfd') -> Gain1/1
  control1/1 -> three-phase active rectifier Voltage Mode/2
  Permanent Magnet Synchronous Generator1/1 -> three-phase active rectifier Voltage Mode/1
  RPM_to_radps/1 -> Permanent Magnet Synchronous Generator1/2, Generator/2(w), Scope2/1
  Sum/1 -> engine torque/1
  Bus Creator/1 -> data_sink/1
  Demux/1 -> Bus Creator1/1  "vd"
  Demux/2 -> Bus Creator1/2  "vq"
  Demux/3 -> Bus Creator1/3  "v0"
  Bus Creator1/1 -> Bus Creator/1  "vdq0 (V)"
  engine speed/1 -> RPM_to_radps/1
  [R_temp_delta] -> Generator/4(Temp)

== system Boeing787_OldMission_ElectricalThermalHydraulicFuelECS/Electrical/Generation Unit Sync-Sync5 ==
  engine speed : Inport
  idq0 : Inport  Port=2
  Temperature : Inport  Port=3
  Bus Creator : BusCreator  Inputs=3
  Bus Creator1 : BusCreator  Inputs=3
  Coeff of Resistance : Gain  Gain=3.85e-3
  Demux : Demux  Outputs=3
  Gain : Gain  Gain=200*2/3
  Gain1 : Gain  Gain=200
  Generator : Subsystem
      mask Display:
      | p = 0:0.1:(2*pi+0.1);
      | plot(sin(p), cos(p));
      | p1 = (-pi/8-0.1-0.2):0.1:(pi/8+0.1-0.2);
      | plot(0.8*sin(p1), 0.8*cos(p1), 0.8*sin(p1+pi), 0.8*cos(p1+pi));
      | p2 = sin((-pi/8-0.1-0.2+pi/8+0.1-0.2)/2);
      | p3 = sin((-pi/8-0.1-0.2+pi/8+0.1-0.2)/2+pi);
      | p4 = cos((-pi/8-0.1-0.2+pi/8+0.1-0.2)/2);
      | p5 = cos((-pi/8-0.1-0.2+pi/8+0.1-0.2)/2+pi);
      | plot(0.8*[p2, p3], 0.8*[p4, p5]);
      | port_label('output', 1, 'Vdq0');
      | port_label('output', 2, 'Te');
      | port_label('output', 3, 'Vfd');
      | port_label('output', 4, 'Ploss');
      | port_label('input', 1, 'idq0');
      | port_label('input', 2, 'w');
      | port_label('input', 3, 'ifd');
  Initial Temperature : Constant  Value=25
  Memory : Memory
  Permanent Magnet Synchronous Generator1 : PowerFlowLib/Energy & Power Systems/Electrical/Machines/Permanent Magnet Synchronous Generator1
  RPM_to_radps : Gain  Gain=pi/30
  Scope2 : Scope
      settings: TimeRange=100  YMin=0  YMax=5500
  Sum : Sum  Inputs=++|
  Sum1 : Sum
  Sum5 : Sum  Inputs=|+-
  Sum6 : Sum  Inputs=|++
  control1 : Constant
  data_sink : PowerFlowLib/Support Functions//Tools/data_sink
  one : Constant
  three-phase active rectifier Voltage Mode : PowerFlowLib/Energy & Power Systems/Electrical/Rectifiers/three-phase  active rectifier Voltage Mode  L=1  C=1e-4
  vdq0 : Outport
  engine torque : Outport  Port=2
  Ploss : Outport  Port=3
  wires:
  Temperature/1 -> Sum5/1
  Initial Temperature/1 -> Sum5/2
  Sum5/1 -> Coeff of Resistance/1
  Coeff of Resistance/1 -> Sum6/1
  one/1 -> Sum6/2
  Sum6/1 -> [R_temp_delta]
  Memory/1 -> Permanent Magnet Synchronous Generator1/1
  Sum1/1 -> Ploss/1, Bus Creator/2  "Ploss (W)"
  Generator/4(Ploss) -> Sum1/2
  Permanent Magnet Synchronous Generator1/3 -> Sum1/1
  Generator/1(vdq0) -> vdq0/1, Demux/1  "Vdq0 (V)"
  idq0/1 -> Generator/1(idq0)
  Generator/2(Te) -> Sum/2
  Permanent Magnet Synchronous Generator1/2 -> Sum/1
  three-phase active rectifier Voltage Mode/2 -> Memory/1
  three-phase active rectifier Voltage Mode/1 -> Gain/1
  Gain/1 -> Bus Creator/3, Generator/3(ifd')  "Excit current (A)"
  Gain1/1 -> three-phase active rectifier Voltage Mode/3
  Generator/3(vfd') -> Gain1/1
  control1/1 -> three-phase active rectifier Voltage Mode/2
  Permanent Magnet Synchronous Generator1/1 -> three-phase active rectifier Voltage Mode/1
  RPM_to_radps/1 -> Permanent Magnet Synchronous Generator1/2, Generator/2(w), Scope2/1
  Sum/1 -> engine torque/1
  Bus Creator/1 -> data_sink/1
  Demux/1 -> Bus Creator1/1  "vd"
  Demux/2 -> Bus Creator1/2  "vq"
  Demux/3 -> Bus Creator1/3  "v0"
  Bus Creator1/1 -> Bus Creator/1  "vdq0 (V)"
  engine speed/1 -> RPM_to_radps/1
  [R_temp_delta] -> Generator/4(Temp)
